simulink subsystem "Subsistema_Termico"  (R2023b)
settings: Solver=VariableStepAuto  StartTime=0.0  StopTime=10.0  RelTol=1e-3
values from neighbouring files (symbols this model uses):
  alfa_Cu = 3.9e-3    (= 0.0039)    [constantes.m]
  C_ts = 0.818    [constantes.m]
  R_sREF = 1.02    [constantes.m]
  R_ts_amb = 146.7    [constantes.m]
  T_s_inicial = 40    [constantes.m]
  T_sREF = 20    [constantes.m]
settings Model: Creator=rodri  LastModifiedBy=nahue

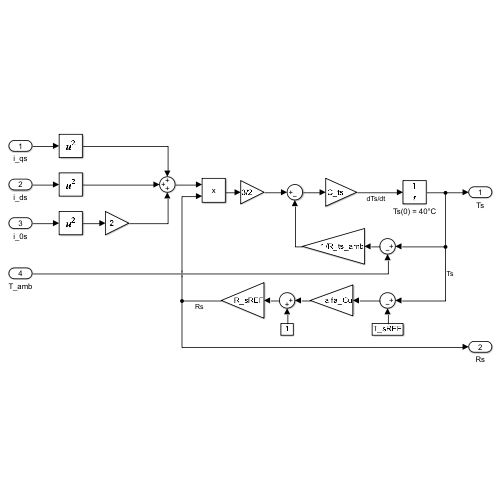
[thumbnail: Simulink's stored preview of the top-level diagram]
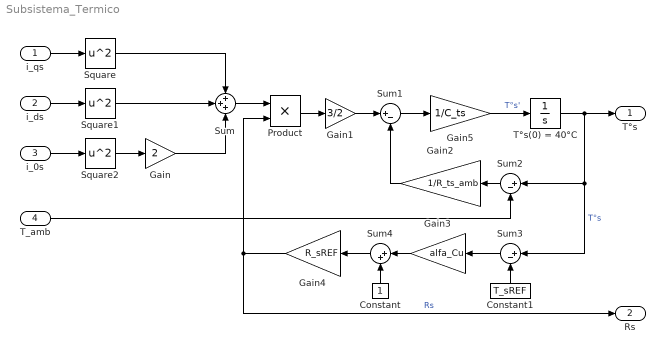
== system Subsistema_Termico ==
  i_qs : Inport
  i_ds : Inport  Port=2
  i_0s : Inport  Port=3
  T_amb : Inport  Port=4
  Constant : Constant
  Constant1 : Constant  Value=T_sREF
  Gain : Gain  Gain=2
  Gain1 : Gain  Gain=3/2
  Gain2 : Gain  Gain=1/R_ts_amb
  Gain3 : Gain  Gain=alfa_Cu
  Gain4 : Gain  Gain=R_sREF
  Gain5 : Gain  Gain=1/C_ts
  Product : Product
  Square : Math  Operator=square
  Square1 : Math  Operator=square
  Square2 : Math  Operator=square
  Sum : Sum  Inputs=+++
  Sum1 : Sum  Inputs=|+-
  Sum2 : Sum  Inputs=|+-
  Sum3 : Sum  Inputs=|+-
  Sum4 : Sum  Inputs=|++
  T°s(0) = 40°C : Integrator  InitialCondition=T_s_inicial
  T°s : Outport
  Rs : Outport  Port=2
  wires:
  i_qs/1 -> Square/1
  i_ds/1 -> Square1/1
  i_0s/1 -> Square2/1
  Square2/1 -> Gain/1
  Square1/1 -> Sum/2
  Square/1 -> Sum/1
  Gain/1 -> Sum/3
  Sum/1 -> Product/1
  Gain4/1 -> Rs/1, Product/2  "Rs"
  Product/1 -> Gain1/1
  Sum1/1 -> Gain5/1
  T°s(0) = 40°C/1 -> T°s/1, Sum2/1, Sum3/1  "T°s"
  T_amb/1 -> Sum2/2
  Sum2/1 -> Gain2/1
  Gain2/1 -> Sum1/2
  Constant1/1 -> Sum3/2
  Sum3/1 -> Gain3/1
  Gain3/1 -> Sum4/1
  Constant/1 -> Sum4/2
  Sum4/1 -> Gain4/1
  Gain5/1 -> T°s(0) = 40°C/1  "T°s'"
  Gain1/1 -> Sum1/1
